simulink model "mpc_rtwdemo"  (Simulink 6.0)
settings: Solver=ode3  SolverMode=SingleTasking  StartTime=0.0  StopTime=Tstop  RelTol=1e-3
values from neighbouring files (symbols this model uses):
  A = sys.a    [misosim.m]    (also in misoss.m)
  B = sys.b    [misosim.m]    (also in misoss.m)
  C = sys.c    [misosim.m]    (also in misoss.m)
  D = sys.d    [misosim.m]    (also in misoss.m)
  x0 = [0 0 0 0 0]'    [misosim.m]    (also in misoss.m; mpcmotormodel.m = zeros(4,1))
libraries: mpclib x1
settings Model: Creator=jowen  LastModifiedBy=rsingh  ExtModeTrigMode=oneshot  ExtModeArmWhenConnect=off
settings DataIOCC: LimitDataPoints=off  SignalLoggingName=sigsOut
settings OptimizationCC: BooleanDataType=off
settings DebuggingCC: CheckExecutionContextPreStartOutputMsg=on  CheckExecutionContextRuntimeOutputMsg=on  SolverPrmCheckMsg=none  IntegerOverflowMsg=none
settings HardwareCC: TargetHWDeviceType=32-bit Generic  ProdEqTarget=off

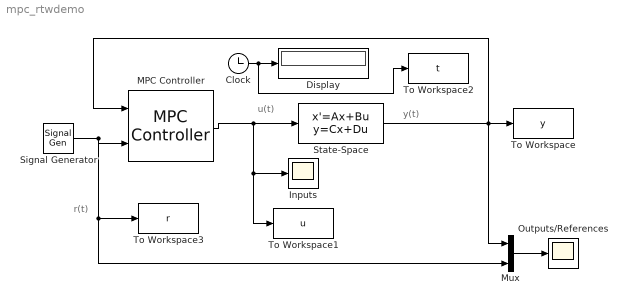
== system mpc_rtwdemo ==
  note: u(t)
  note: y(t)
  note: r(t)
  Clock : Clock
      settings: Decimation=10
  Display : Display
  Inputs : Scope
      settings: TimeRange=10  YMin=-1.5  YMax=1.5  DataFormat=Structure
  MPC Controller : mpclib/MPC Controller  mpcobj=mpccon  n_mv=0  x0=[]  ref_from_ws=off  ref_signal_name=[]  ref_preview=on  md_from_ws=off  md_signal_name=[]  md_preview=on  from_project=off  md_inport=off  project_file=MPCtask.mat
  Mux : Mux  Inputs=2
  Outputs/References : Scope
      settings: TimeRange=10  YMin=-1  YMax=1  DataFormat=Structure
  Signal Generator : SignalGenerator  Frequency=.4
  State-Space : StateSpace  A=A  B=B  C=C  D=D  X0=x0
  To Workspace : ToWorkspace  VariableName=y  SampleTime=-1  SaveFormat=Array
      settings: MaxDataPoints=Inf
  To Workspace1 : ToWorkspace  VariableName=u  SampleTime=-1  SaveFormat=Array
      settings: MaxDataPoints=Inf
  To Workspace2 : ToWorkspace  VariableName=t  SampleTime=-1  SaveFormat=Array
      settings: MaxDataPoints=Inf
  To Workspace3 : ToWorkspace  VariableName=r  SampleTime=-1  SaveFormat=Array
      settings: MaxDataPoints=Inf
  wires:
  MPC Controller/1 -> State-Space/1, Inputs/1, To Workspace1/1
  State-Space/1 -> To Workspace/1, Mux/1, MPC Controller/1
  Mux/1 -> Outputs/References/1
  Signal Generator/1 -> Mux/2, To Workspace3/1, MPC Controller/2
  Clock/1 -> Display/1, To Workspace2/1
